simulink model "Pos_CBAgent"  (Simulink 7.1)
settings: Solver=ode45  SolverMode=SingleTasking  StartTime=0.0  StopTime=10.0  RelTol=1e-3  AbsTol=1e-6
settings Model: Creator=The MathWorks Inc.  LastModifiedBy=suarezjl  ExtModeTrigMode=oneshot  ExtModeArmWhenConnect=off  ExtModeAutoUpdateStatusClock=off
settings DataIOCC: LimitDataPoints=off  SignalLoggingName=logsOut
settings OptimizationCC: BooleanDataType=off  InlineInvariantSignals=on
settings DebuggingCC: SaveWithParameterizedLinksMsg=none  CheckExecutionContextPreStartOutputMsg=on  CheckExecutionContextRuntimeOutputMsg=on  SignalResolutionControl=TryResolveAllWithWarning  SolverPrmCheckMsg=none  MultiTaskDSMMsg=warning  MultiTaskCondExecSysMsg=none  IntegerOverflowMsg=none  StrictBusMsg=None
settings HardwareCC: TargetUnknown=on
settings ModelReferenceCC: UpdateModelReferenceTargets=IfOutOfDate
settings RTWCC: IncludeERTFirstTime=on
settings GRTTargetCC: TargetFcnLib=ansi_tfl_tmw.mat

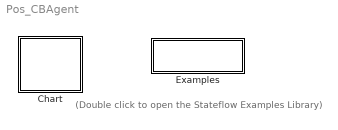
== system Pos_CBAgent ==
  note: (Double click to open the
      | Stateflow Examples Library)
  Chart : Stateflow chart
  Examples : Subsystem
      settings: OpenFcn=sf('Private','sf_examples')
      mask Display: disp('Examples')

== system Pos_CBAgent/Examples ==

== stateflow chart Chart ==
  state Initialize
    \\Octavia\ISACControlBasisModule\RightModule\Arm\ArmController.DoHomingRoutine()
    \\Octavia\ISACControlBasisModule\PosCB\StateMachine.Wait(5000)
    \\Octavia\ISACControlBasisModule\LeftModule\Arm\ArmController.DoHomingRoutine()
    \\Octavia\ISACControlBasisModule\PosCB\StateMachine.Wait(5000)
    \\Octavia\ISACControlBasisModule\PosCB\FKinLeft.Initialize()
    \\Octavia\ISACControlBasisModule\PosCB\FkinRight.Initialize()
    \\Octavia\ISACControlBasisModule\PosCB\PosCBLeft.Initialize()
    \\Octavia\ISACControlBasisModule\PosCB\PosCBRight.Initialize()
  state ControlBasis
    \\Octavia\ISACControlBasisModule\RightModule\Arm\ArmController.Move()
    \\Octavia\ISACControlBasisModule\LeftModule\Arm\ArmController.Move()
    \\Octavia\ISACControlBasisModule\PosCB\FKinLeft.kin_ForwardKinematics()
    \\Octavia\ISACControlBasisModule\PosCB\FkinRight.kin_ForwardKinematics()
    \\Octavia\ISACControlBasisModule\PosCB\PosCBLeft.ComputeControlBasis()
    \\Octavia\ISACControlBasisModule\PosCB\PosCBRight.ComputeControlBasis()
  state End
    \\Octavia\ISACControlBasisModule\PosCB\PosCBLeft.Close()
    \\Octavia\ISACControlBasisModule\PosCB\PosCBRight.Close()
  (default) -> Initialize : Start
  Initialize -> ControlBasis : Signal="Next"
  ControlBasis -> ControlBasis [order 1] : Default
  ControlBasis -> End [order 2] : Signal="Next"
